simulink model "test"  (Simulink 5.0)
settings: Solver=ode4  StartTime=0.0  StopTime=Inf  RelTol=1e-3
undefined symbols (not defined in the file): rtai_lib, Scope
settings Model: Creator=bucher  LastModifiedBy=bucher  ExtModeTrigMode=oneshot  ExtModeArmWhenConnect=off  ExtModeAutoUpdateStatusClock=off  LimitDataPoints=off  BooleanDataType=off  RTWSystemTargetFile=krtai.tlc  RTWTemplateMakefile=krtai.tmf  RTWOptions="-aEnforceIntegerDowncast=1 -aExtMode=0 -aFoldNonRolledExpr=1 -aForceParamTrailComments=0 -aGenerateComments=1 -aGenerateReport=0 -aIncDataTypeInIds=0 -aIncHierarchyInIds=0 -aInlineInvariantSignals=0 -aInlineParameters=0 -aInlinedPrmAccess=\"Literals\" -aLocalBlockOutputs=1 -aLogVarNameModifier=\"rt_\" -aMaxRTWIdLen=31 -aPrefixModelToSubsysFcnNames=1 -aRTWVerbose=1 -aRollThreshold=5 -aShowEliminatedStatements=1"

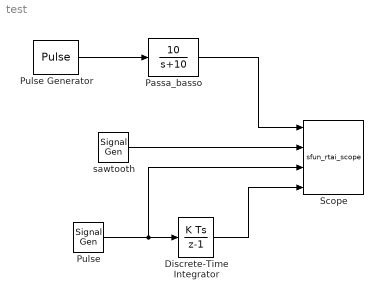
== system test ==
  Discrete-Time Integrator : DiscreteIntegrator  SampleTime=0.001
  Passa_basso : TransferFcn  Numerator=[10]  Denominator=[1 10]
  Pulse : SignalGenerator  WaveForm=square  Frequency=1.2
  Pulse Generator : DiscretePulseGenerator  Amplitude=2  Period=10000  PulseWidth=5000  SampleTime=0.001
  Scope : S-Function  AncestorBlock=rtai_lib/Scope  FunctionName=sfun_rtai_scope  Parameters=numch,ts  mask{numch=4, ts=0.001}
      mask prompts: numch "Channels:"; ts "Sampling Time"
      mask StyleString: popup(1|2|3|4|5|6),edit
  sawtooth : SignalGenerator  WaveForm=sawtooth
  wires:
  Pulse Generator/1 -> Passa_basso/1
  sawtooth/1 -> Scope/2
  Pulse/1 -> Discrete-Time Integrator/1, Scope/3
  Discrete-Time Integrator/1 -> Scope/4
  Passa_basso/1 -> Scope/1
